simulink model "AdaptiveSync_2_4"  (R2016a)
settings: Solver=ode23tb  SolverMode=SingleTasking  StartTime=0.0  StopTime=25  MaxStep=0.01  RelTol=1e-3
values from neighbouring files (symbols this model uses):
  A1obs = [0 -2;1 -1]    [Adaptive_Synchronization.m]
  A2obs = [0 -2.5;1 -0.5]    [Adaptive_Synchronization.m]
  A3obs = [0 -2;1 -1.25]    [Adaptive_Synchronization.m]
  A4obs = [0 -1;1 -0.5]    [Adaptive_Synchronization.m]
  A5obs = [0 -1;1 -0.75]    [Adaptive_Synchronization.m]
  Am = [0 1;-(0.7)^2, 0]    [Adaptive_Synchronization.m]
  B1obs = [1.5;1]    [Adaptive_Synchronization.m]
  B2obs = [1;0.5]    [Adaptive_Synchronization.m]
  B3obs = [1;1.25]    [Adaptive_Synchronization.m]
  B4obs = [0.75;0.75]    [Adaptive_Synchronization.m]
  B5obs = [2;1.5]    [Adaptive_Synchronization.m]
  Bm = [0;1]    [Adaptive_Synchronization.m]
  C1obs = [0 1]    [Adaptive_Synchronization.m]
  C2obs = [0 1]    [Adaptive_Synchronization.m]
  C3obs = [0 1]    [Adaptive_Synchronization.m]
  C4obs = [0 1]    [Adaptive_Synchronization.m]
  C5obs = [0 1]    [Adaptive_Synchronization.m]
  Filterpole = -1    [Adaptive_Synchronization.m]
  L = [1,[-1;0;0;0;0]';[-1;0;0;0;0],(diag([4 2 3 2 2])-Adj)]    [Adaptive_Synchronization.m]
  MRACgam1 = 2000    [Adaptive_Synchronization.m]
  MRACgam2 = 2000    [Adaptive_Synchronization.m]
  MRACgam3 = 2000    [Adaptive_Synchronization.m]
  MRACgam4 = 2000    [Adaptive_Synchronization.m]
  MRACgam5 = 2000    [Adaptive_Synchronization.m]
  x01 = [-0.5;1]    [Adaptive_Synchronization.m]
  x02 = [0.5;-1]    [Adaptive_Synchronization.m]
  x03 = [1;0.5]    [Adaptive_Synchronization.m]
  x04 = [-1;-0.5]    [Adaptive_Synchronization.m]
  x05 = [0;0]    [Adaptive_Synchronization.m]
  x0m = [0;1]    [Adaptive_Synchronization.m]
settings Model: Creator=danielvos  LastModifiedBy=danielvos
settings SolverCC: ZeroCrossAlgorithm=Adaptive
settings DebuggingCC: SFUnexpectedBacktrackingDiag=error  SFNoUnconditionalDefaultTransitionDiag=error
settings GRTTargetCC: TargetLangStandard=C99 (ISO)  GeneratePreprocessorConditionals=Use local settings
settings ConfigComp: CovMetricSettings=dwe  CovHtmlReporting=off  CovSaveCumulativeToWorkspaceVar=off  CovSaveSingleToWorkspaceVar=off  CovExternalEMLEnable=on

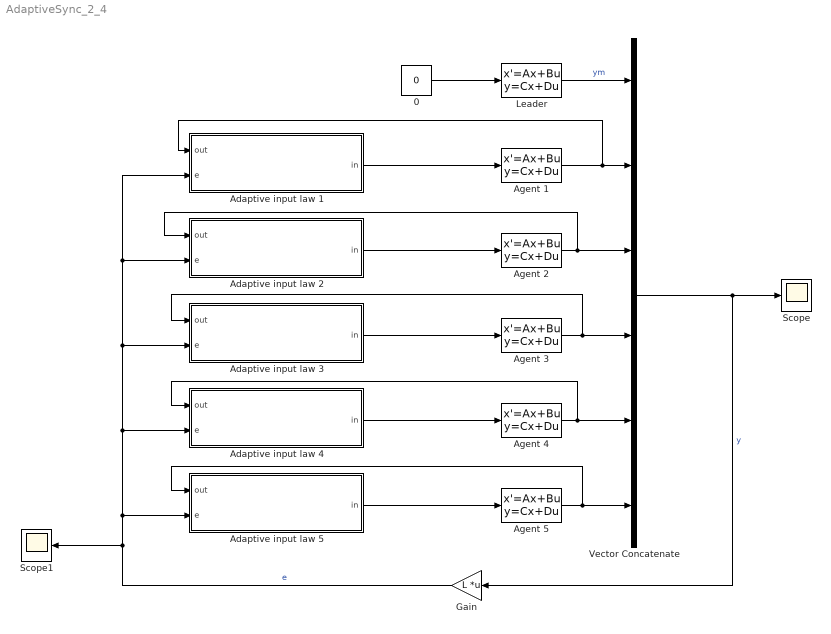
== system AdaptiveSync_2_4 ==
  0 : Constant  Value=0
  Adaptive input law 1 : Subsystem
  Adaptive input law 2 : Subsystem
  Adaptive input law 3 : Subsystem
  Adaptive input law 4 : Subsystem
  Adaptive input law 5 : Subsystem
  Agent 1 : StateSpace  A=A1obs  B=B1obs  C=C1obs  D=0  X0=x01
  Agent 2 : StateSpace  A=A2obs  B=B2obs  C=C2obs  D=0  X0=x02
  Agent 3 : StateSpace  A=A3obs  B=B3obs  C=C3obs  D=0  X0=x03
  Agent 4 : StateSpace  A=A4obs  B=B4obs  C=C4obs  D=0  X0=x04
  Agent 5 : StateSpace  A=A5obs  B=B5obs  C=C5obs  D=0  X0=x05
  Gain : Gain  Gain=L  Multiplication=Matrix(K*u)
  Leader : StateSpace  A=Am  B=Bm  C=[0 1]  D=0  X0=x0m
  Scope : Scope
  Scope1 : Scope
  Vector Concatenate : Concatenate  NumInputs=6
  wires:
  Leader/1 -> Vector Concatenate/1  "ym"
  0/1 -> Leader/1
  Agent 1/1 -> Adaptive input law 1/1(out), Vector Concatenate/2
  Agent 2/1 -> Adaptive input law 2/1(out), Vector Concatenate/3
  Agent 3/1 -> Adaptive input law 3/1(out), Vector Concatenate/4
  Agent 4/1 -> Adaptive input law 4/1(out), Vector Concatenate/5
  Agent 5/1 -> Adaptive input law 5/1(out), Vector Concatenate/6
  Vector Concatenate/1 -> Scope/1, Gain/1  "y"
  Gain/1 -> Adaptive input law 4/2(e), Adaptive input law 3/2(e), Adaptive input law 2/2(e), Adaptive input law 1/2(e), Adaptive input law 5/2(e), Scope1/1  "e"
  Adaptive input law 1/1(in) -> Agent 1/1
  Adaptive input law 2/1(in) -> Agent 2/1
  Adaptive input law 3/1(in) -> Agent 3/1
  Adaptive input law 4/1(in) -> Agent 4/1
  Adaptive input law 5/1(in) -> Agent 5/1

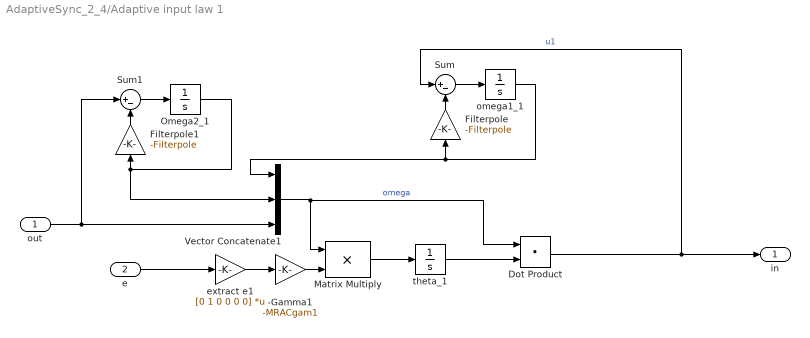
== system AdaptiveSync_2_4/Adaptive input law 1 ==
  out : Inport
  e : Inport  Port=2
  -Gamma1 : Gain  Gain=-MRACgam1
  Dot Product : DotProduct  InputSameDT=on  OutDataTypeStr=Inherit: Inherit via internal rule
  Filterpole : Gain  Gain=-Filterpole
  Filterpole1 : Gain  Gain=-Filterpole
  Matrix Multiply : Product
  Omega2_1 : Integrator  InitialCondition=1
  Sum : Sum  Inputs=|+-
  Sum1 : Sum  Inputs=|+-
  Vector Concatenate1 : Concatenate  NumInputs=3
  extract e1 : Gain  Gain=[0 1 0 0 0 0]  Multiplication=Matrix(K*u)
  omega1_1 : Integrator  InitialCondition=1
  theta_1 : Integrator  InitialCondition=[1;1;1]
  in : Outport
  wires:
  e/1 -> extract e1/1
  Sum/1 -> omega1_1/1
  theta_1/1 -> Dot Product/2
  -Gamma1/1 -> Matrix Multiply/2
  Vector Concatenate1/1 -> Matrix Multiply/1, Dot Product/1  "omega"
  Matrix Multiply/1 -> theta_1/1
  Dot Product/1 -> in/1, Sum/1  "u1"
  extract e1/1 -> -Gamma1/1
  Sum1/1 -> Omega2_1/1
  Omega2_1/1 -> Vector Concatenate1/2, Filterpole1/1
  omega1_1/1 -> Filterpole/1, Vector Concatenate1/1
  out/1 -> Sum1/1, Vector Concatenate1/3
  Filterpole/1 -> Sum/2
  Filterpole1/1 -> Sum1/2

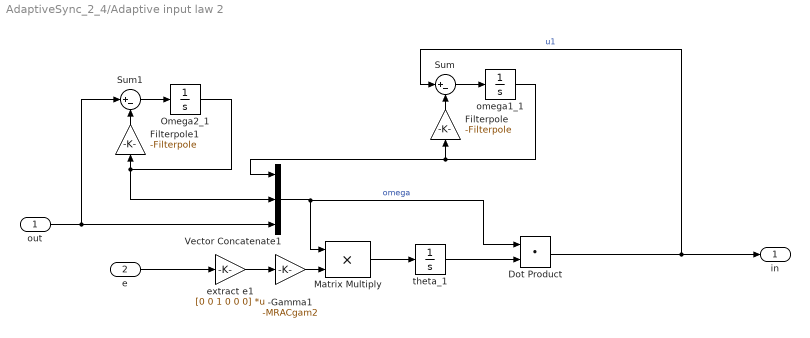
== system AdaptiveSync_2_4/Adaptive input law 2 ==
  out : Inport
  e : Inport  Port=2
  -Gamma1 : Gain  Gain=-MRACgam2
  Dot Product : DotProduct  InputSameDT=on  OutDataTypeStr=Inherit: Inherit via internal rule
  Filterpole : Gain  Gain=-Filterpole
  Filterpole1 : Gain  Gain=-Filterpole
  Matrix Multiply : Product
  Omega2_1 : Integrator  InitialCondition=1
  Sum : Sum  Inputs=|+-
  Sum1 : Sum  Inputs=|+-
  Vector Concatenate1 : Concatenate  NumInputs=3
  extract e1 : Gain  Gain=[0 0 1 0 0 0]  Multiplication=Matrix(K*u)
  omega1_1 : Integrator  InitialCondition=1
  theta_1 : Integrator  InitialCondition=[1;1;1]
  in : Outport
  wires:
  e/1 -> extract e1/1
  Sum/1 -> omega1_1/1
  theta_1/1 -> Dot Product/2
  -Gamma1/1 -> Matrix Multiply/2
  Vector Concatenate1/1 -> Matrix Multiply/1, Dot Product/1  "omega"
  Matrix Multiply/1 -> theta_1/1
  Dot Product/1 -> in/1, Sum/1  "u1"
  extract e1/1 -> -Gamma1/1
  Sum1/1 -> Omega2_1/1
  Omega2_1/1 -> Filterpole1/1, Vector Concatenate1/2
  omega1_1/1 -> Filterpole/1, Vector Concatenate1/1
  out/1 -> Sum1/1, Vector Concatenate1/3
  Filterpole/1 -> Sum/2
  Filterpole1/1 -> Sum1/2

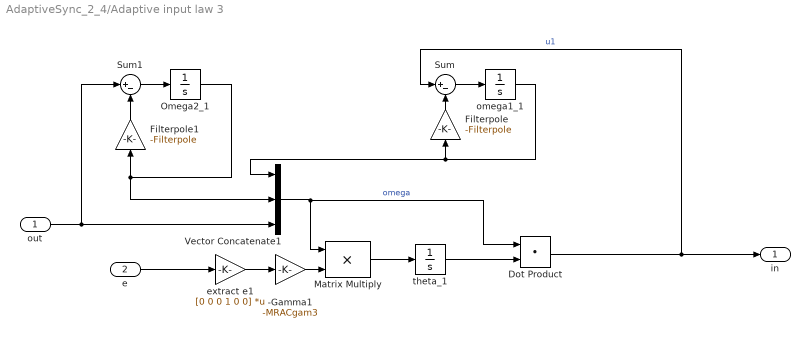
== system AdaptiveSync_2_4/Adaptive input law 3 ==
  out : Inport
  e : Inport  Port=2
  -Gamma1 : Gain  Gain=-MRACgam3
  Dot Product : DotProduct  InputSameDT=on  OutDataTypeStr=Inherit: Inherit via internal rule
  Filterpole : Gain  Gain=-Filterpole
  Filterpole1 : Gain  Gain=-Filterpole
  Matrix Multiply : Product
  Omega2_1 : Integrator  InitialCondition=1
  Sum : Sum  Inputs=|+-
  Sum1 : Sum  Inputs=|+-
  Vector Concatenate1 : Concatenate  NumInputs=3
  extract e1 : Gain  Gain=[0 0 0 1 0 0]  Multiplication=Matrix(K*u)
  omega1_1 : Integrator  InitialCondition=1
  theta_1 : Integrator  InitialCondition=[1;1;1]
  in : Outport
  wires:
  e/1 -> extract e1/1
  Sum/1 -> omega1_1/1
  theta_1/1 -> Dot Product/2
  -Gamma1/1 -> Matrix Multiply/2
  Vector Concatenate1/1 -> Matrix Multiply/1, Dot Product/1  "omega"
  Matrix Multiply/1 -> theta_1/1
  Dot Product/1 -> in/1, Sum/1  "u1"
  extract e1/1 -> -Gamma1/1
  Sum1/1 -> Omega2_1/1
  Omega2_1/1 -> Vector Concatenate1/2, Filterpole1/1
  omega1_1/1 -> Filterpole/1, Vector Concatenate1/1
  out/1 -> Sum1/1, Vector Concatenate1/3
  Filterpole/1 -> Sum/2
  Filterpole1/1 -> Sum1/2

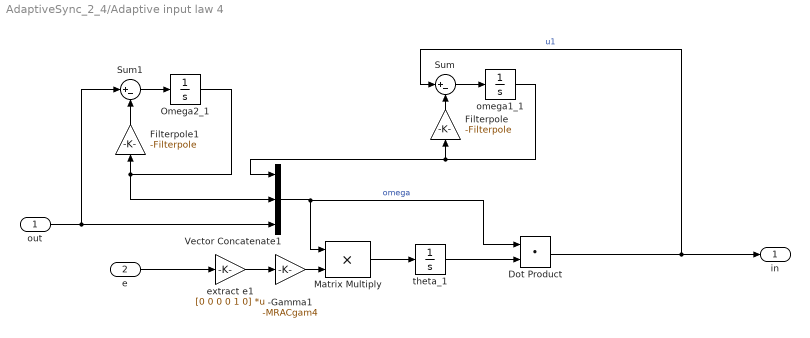
== system AdaptiveSync_2_4/Adaptive input law 4 ==
  out : Inport
  e : Inport  Port=2
  -Gamma1 : Gain  Gain=-MRACgam4
  Dot Product : DotProduct  InputSameDT=on  OutDataTypeStr=Inherit: Inherit via internal rule
  Filterpole : Gain  Gain=-Filterpole
  Filterpole1 : Gain  Gain=-Filterpole
  Matrix Multiply : Product
  Omega2_1 : Integrator  InitialCondition=1
  Sum : Sum  Inputs=|+-
  Sum1 : Sum  Inputs=|+-
  Vector Concatenate1 : Concatenate  NumInputs=3
  extract e1 : Gain  Gain=[0 0 0 0 1 0]  Multiplication=Matrix(K*u)
  omega1_1 : Integrator  InitialCondition=1
  theta_1 : Integrator  InitialCondition=[1;1;1]
  in : Outport
  wires:
  e/1 -> extract e1/1
  Sum/1 -> omega1_1/1
  theta_1/1 -> Dot Product/2
  -Gamma1/1 -> Matrix Multiply/2
  Vector Concatenate1/1 -> Matrix Multiply/1, Dot Product/1  "omega"
  Matrix Multiply/1 -> theta_1/1
  Dot Product/1 -> in/1, Sum/1  "u1"
  extract e1/1 -> -Gamma1/1
  Sum1/1 -> Omega2_1/1
  Omega2_1/1 -> Vector Concatenate1/2, Filterpole1/1
  omega1_1/1 -> Filterpole/1, Vector Concatenate1/1
  out/1 -> Sum1/1, Vector Concatenate1/3
  Filterpole/1 -> Sum/2
  Filterpole1/1 -> Sum1/2

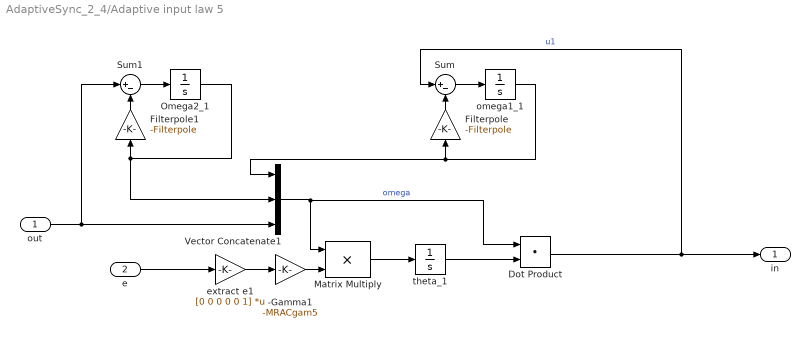
== system AdaptiveSync_2_4/Adaptive input law 5 ==
  out : Inport
  e : Inport  Port=2
  -Gamma1 : Gain  Gain=-MRACgam5
  Dot Product : DotProduct  InputSameDT=on  OutDataTypeStr=Inherit: Inherit via internal rule
  Filterpole : Gain  Gain=-Filterpole
  Filterpole1 : Gain  Gain=-Filterpole
  Matrix Multiply : Product
  Omega2_1 : Integrator  InitialCondition=1
  Sum : Sum  Inputs=|+-
  Sum1 : Sum  Inputs=|+-
  Vector Concatenate1 : Concatenate  NumInputs=3
  extract e1 : Gain  Gain=[0 0 0 0 0 1]  Multiplication=Matrix(K*u)
  omega1_1 : Integrator  InitialCondition=1
  theta_1 : Integrator  InitialCondition=[1;1;1]
  in : Outport
  wires:
  e/1 -> extract e1/1
  Sum/1 -> omega1_1/1
  theta_1/1 -> Dot Product/2
  -Gamma1/1 -> Matrix Multiply/2
  Vector Concatenate1/1 -> Matrix Multiply/1, Dot Product/1  "omega"
  Matrix Multiply/1 -> theta_1/1
  Dot Product/1 -> in/1, Sum/1  "u1"
  extract e1/1 -> -Gamma1/1
  Sum1/1 -> Omega2_1/1
  Omega2_1/1 -> Vector Concatenate1/2, Filterpole1/1
  omega1_1/1 -> Filterpole/1, Vector Concatenate1/1
  out/1 -> Sum1/1, Vector Concatenate1/3
  Filterpole/1 -> Sum/2
  Filterpole1/1 -> Sum1/2
